simulink model "EcoSIM3_P2_C2_WIP"  (R2014b)
settings: Solver=ode1  SolverMode=SingleTasking  StartTime=0.0  StopTime=inf  FixedStep=0.01  RelTol=1e-3
PostLoadFcn:
  | %, if any(exist('dsrtsu_mdlpostloadfcn', 'file') == [2, 3, 6]), try dsrtsu_mdlpostloadfcn('Execute', bdroot); catch fprintf('Error in PostLoadFcn (dsrtsu_mdlpostloadfcn) for model "%s":\n %s\n', bdroot, lasterr); end, end,
InitFcn:
  | tic
  | %Startup_EcoSIM
values from neighbouring files (symbols this model uses):
  EngPwr = [0 5	10	15	20	25	30	35	40	45	50	55	60	65	70	75	80	85	90	95	100	105	110	115]    [Series_Maps.m]
  EngSpd = [0 477.4645 954.929 1909.858 2864.787 3819.716 4774.645 5729.574 6684.503]    [Series_Maps.m]
  EngTrq = [0	0	0	0	0	0	0	0	0	0	0	0	0	0	0	0	0	0	0	0	0	0	0	0 ... (first row only)    [Series_Maps.m]
  Power = [0 5 10 15 20 25 30]    [Series_Maps.m]
  Torque = [-50,-40,-30,-25,-20,-15,-10,-8,-6,-4,-2,0]    [Series_Maps.m]
undefined symbols (not defined in the file or in its folder): canChannel, Controls, DriveCycles, Driver, EM_EFF_MAP, EM_PwrLoss_MAP, Glbl, Overwritten_Mode, Plants, sigbuilder_block, Trialmap, Veh_Dynamics
libraries: simulink x141, canmsglib x113, fl_lib x104, canlib x89, nesl_utility x56, sdl_lib x29, dspsigops x6, dspswit3 x5, dspstat3 x2, commnoisgen2 x1, dspfdesign x1
(part 3 of 21)

== system EcoSIM3_P2_C2_WIP/Powertrain/Accessories Power Module/Plant ==
  Actuator_Cmds : Inport
  Bus Creator1 : BusCreator  Inputs=2
  Bus Creator2 : BusCreator  Inputs=2
  Bus Creator3 : BusCreator  Inputs=3
  Bus Selector : BusSelector  OutputSignals=Accessories_Power_In_W,AccPwrMdlLowVlt,Accessories_Power_In_W,bcm_vbat
  Chart : Stateflow chart  Commented=on  TreatAsAtomicUnit=on
  Constant : Constant  Value=0
  Constant1 : Constant  Value=0
  Constant2 : Constant  Value=25
  Constant3 : Constant  Value=25
  Constant4 : Constant  Value=0
  DCDC_Eff : Gain  Gain=1/Plants.DCDC.Eff
  Data Type Conversion2 : DataTypeConversion  OutDataTypeStr=boolean
  Divide : Product  Inputs=*/
  Divide1 : Product  Inputs=*/
  Saturation1 : Saturate  UpperLimit=255  LowerLimit=0
  Switch : Switch  Criteria=u2 > Threshold
  Switch1 : Switch  Criteria=u2 > Threshold
  Sensor_Out : Outport
  tag scope: DCDC_HV_Crnt=global
  wires:
  Constant4/1 -> Data Type Conversion2/1
  Data Type Conversion2/1 -> Bus Creator3/3  "Fault"
  Constant3/1 -> Bus Creator3/2  "AccPwrModTmp2"
  Constant2/1 -> Bus Creator3/1  "AccPwrModTmp1"
  Bus Creator3/1 -> Bus Creator2/1  "Temperature_Sensors"
  Bus Creator1/1 -> Bus Creator2/2  "Electrical_Sensors"
  Bus Creator2/1 -> Sensor_Out/1  "APM_Sensor_Out"
  Actuator_Cmds/1 -> Bus Selector/1
  Bus Selector/2 -> Divide/2, Switch/2  "<AccPwrMdlLowVlt>"
  Switch/1 -> Bus Creator1/1  "APMLwVltOtptCrntUns"
  Bus Selector/1 -> Divide/1  "<Accessories_Power_In_W>"
  Bus Selector/4 -> Divide1/2, Switch1/2  "<bcm_vbat>"
  Switch1/1 -> [DCDC_HV_Crnt], Bus Creator1/2  "AccPwrMdlHiVltInpCrnt"
  Divide/1 -> Saturation1/1
  Saturation1/1 -> Switch/1
  Constant/1 -> Switch/3
  Divide1/1 -> DCDC_Eff/1
  DCDC_Eff/1 -> Switch1/1
  Constant1/1 -> Switch1/3
  Bus Selector/3 -> Divide1/1  "<Accessories_Power_In_W>"

== system EcoSIM3_P2_C2_WIP/Powertrain/Accessories Power Module/Subsystem ==
  CAN_In : Inport
  Sensor_In : Inport  Port=2
  Algorithm : Subsystem
  Inputs : Subsystem
  Outputs : Subsystem
  To ECU : Outport
  Actuator_Cmds : Outport  Port=2
  wires:
  CAN_In/1 -> Inputs/1(CAN_In)  "APM_CAN_In"
  Algorithm/1(Outputs) -> Outputs/1(From Algorithm)
  Sensor_In/1 -> Inputs/2(Sensors)
  Inputs/1(To_Algorithm) -> Algorithm/1(Inputs)
  Outputs/1(To ECU) -> To ECU/1
  Outputs/2(Actuator_Cmds) -> Actuator_Cmds/1

== system EcoSIM3_P2_C2_WIP/Powertrain/BAS Motor/ Compnent Model ==
  Actuator_Cmds : Inport
  Actuators : Subsystem
  Plant : Subsystem
  Sensors : Subsystem
  To_Plants : PMIOPort  Port=1  Side=Right
  Sensor_Out : Outport
  To_Battery : Outport  Port=2
  wires:
  Actuator_Cmds/1 -> Actuators/1(ActuatorInputs)
  Actuators/1(Actuator Outputs) -> Plant/1(From_Actuators)
  Sensors/1(Sensor Out) -> Sensor_Out/1, Plant/2(Sensor_Feedback)  "BAS_Sensor_Out"
  Sensors/2(Battery) -> To_Battery/1
  connections:
  To_Plants/RConn1 -- Sensors/RConn1
  Plant/RConn1 -- Sensors/LConn1

== system EcoSIM3_P2_C2_WIP/Powertrain/BAS Motor/BAS_Receive ==
  note: Put the CAN Recieve Block placed in the
      | Vehicle Network ToolBox and define the
      | Messages required
  From_ECUs : Outport
  wires:
  [BAS_SoftECU_Receive] -> From_ECUs/1  "BAS_SoftECU_Receive"

== system EcoSIM3_P2_C2_WIP/Powertrain/BAS Motor/BAS_Transmit ==
  note: Put the CAN Transmit Block placed in the
      | Vehicle Network ToolBox and define the
      | Messages required
  To_ECUs : Inport
  Bus Creator{,1,3..4} (4 alike) : BusCreator  Inputs=2
  Bus Creator2 : BusCreator  Inputs=3
  Bus Selector : BusSelector  OutputSignals=BAS_Speed_rad_per_s,BAS_Torque_Out_Nm,BAS_Torque_Command_Nm,BAS_Status_Mode,BAS_Fault_Status,Fault_U,Fault_V,Fault_W
  Ground : Ground
  Ground1 : Ground
  Terminator : Terminator
  Terminator1 : Terminator
  Terminator2 : Terminator
  tag scope: BAS_SoftECU_Transmit=global
  wires:
  Bus Creator4/1 -> [BAS_SoftECU_Transmit]  "BAS_Transmit"
  To_ECUs/1 -> Bus Selector/1
  Bus Selector/6 -> Bus Creator2/1  "<Fault_U>"
  Bus Selector/3 -> Terminator/1  "<BAS_Torque_Command_Nm>"
  Bus Selector/8 -> Bus Creator2/3  "<Fault_W>"
  Bus Selector/1 -> Bus Creator1/1  "<BAS_Speed_rad_per_s>"
  Bus Selector/4 -> Terminator1/1  "<BAS_Status_Mode>"
  Bus Selector/7 -> Bus Creator2/2  "<Fault_V>"
  Bus Selector/5 -> Terminator2/1  "<BAS_Fault_Status>"
  Bus Creator1/1 -> Bus Creator/1  "Status_1"
  Bus Selector/2 -> Bus Creator1/2  "<BAS_Torque_Out_Nm>"
  Bus Creator2/1 -> Bus Creator/2  "Status_2"
  Bus Creator/1 -> Bus Creator4/1  "BAS_CAN_Out"
  Bus Creator3/1 -> Bus Creator4/2  "BAS_Electrical_Out"
  Ground1/1 -> Bus Creator3/2  "Dummy2"
  Ground/1 -> Bus Creator3/1  "Dummy1"

== system EcoSIM3_P2_C2_WIP/Powertrain/BAS Motor/Soft ECU ==
  CAN_In : Inport
  Sensor_In : Inport  Port=2
  Algorithm : Subsystem
  Inputs : Subsystem
  Inputs1 : Subsystem
  CAN_Out : Outport
  Actuator_Cmds : Outport  Port=2
  wires:
  Sensor_In/1 -> Inputs/2(Sensors)
  CAN_In/1 -> Inputs/1(CAN_In)
  Inputs/1(To_Algorithm) -> Algorithm/1(Inputs)
  Algorithm/1(Outputs) -> Inputs1/1(From Algorithm)
  Inputs1/1(CAN Out) -> CAN_Out/1
  Inputs1/2(Actuator Cmds) -> Actuator_Cmds/1

== system EcoSIM3_P2_C2_WIP/Powertrain/Belt Coupler/Sensors ==
  note: Sensor Model: Place where we add Corrupter
  Ideal Rotational Motion Sensor : fl_lib/Mechanical/Mechanical Sensors/Ideal Rotational Motion Sensor  offset=0 rad
  Ideal Torque Sensor : fl_lib/Mechanical/Mechanical Sensors/Ideal Torque Sensor
  Mechanical Rotational Reference1 : fl_lib/Mechanical/Rotational Elements/Mechanical Rotational Reference
  PS-Simulink Converter : nesl_utility/PS-Simulink Converter  PhysicalDomain=network_engine_domain  SubClassName=ps_output  LeftPortType=input  RightPortType=output  PseudoPeriodic=off  Frequencies=[]  Unit=rad/s  AffineConversion=off
  PS-Simulink Converter1 : nesl_utility/PS-Simulink Converter  PhysicalDomain=network_engine_domain  SubClassName=ps_output  LeftPortType=input  RightPortType=output  PseudoPeriodic=off  Frequencies=[]  Unit=N*m  AffineConversion=off
  Terminator : Terminator
  Terminator1 : Terminator
  Shaft : PMIOPort  Port=1  Side=Left
  To_Clutch : PMIOPort  Tag=PMCPort  Port=2  Side=Right
  wires:
  PS-Simulink Converter/1 -> Terminator/1  "Belt_Speed_rad_per_s"
  PS-Simulink Converter1/1 -> Terminator1/1  "Belt_Torque_Out_Nm"
  connections:
  Ideal Torque Sensor/LConn1 -- Shaft/RConn1 -- Ideal Rotational Motion Sensor/LConn1
  Ideal Rotational Motion Sensor/RConn1 -- Mechanical Rotational Reference1/LConn1
  PS-Simulink Converter/LConn1 -- Ideal Rotational Motion Sensor/RConn2
  PS-Simulink Converter1/LConn1 -- Ideal Torque Sensor/RConn2
  To_Clutch/RConn1 -- Ideal Torque Sensor/RConn1

== system EcoSIM3_P2_C2_WIP/Powertrain/Charger/CAN_Revieve ==
  note: Put the CAN Recieve Block placed in the
      | Vehicle Network ToolBox and define the
      | Messages required
  Bus Selector : BusSelector  OutputSignals=Brusa_Electrical.PON
  From_ECUs : Outport
  wires:
  [Brusa_SoftECU_Receive] -> Bus Selector/1
  Bus Selector/1 -> From_ECUs/1  "<PON>"

== system EcoSIM3_P2_C2_WIP/Powertrain/Charger/CAN_Transmit ==
  note: Put the CAN Transmit Block placed in the
      | Vehicle Network ToolBox and define the
      | Messages required
  To_CAN : Inport
  Bus Creator : BusCreator  Inputs=1
  Bus Creator1 : BusCreator  Inputs=2
  Bus Creator3 : BusCreator  Inputs=1
  Bus Creator4 : BusCreator  Inputs=2
  Bus Selector : BusSelector  OutputSignals=chga_wake,GCM_Wakeup_charge
  Ground : Ground
  Ground1 : Ground
  Terminator : Terminator
  tag scope: Brusa_SoftECU_Transmit=global
  wires:
  To_CAN/1 -> Bus Selector/1
  Bus Creator/1 -> Bus Creator4/1  "Brusa_CAN_Out"
  Bus Creator1/1 -> Bus Creator/1  "Brusa_Dummy_msg"
  Bus Creator3/1 -> Bus Creator4/2  "Brusa_Electrical_Out"
  Bus Creator4/1 -> [Brusa_SoftECU_Transmit]  "Brusa_Transmit"
  Ground1/1 -> Bus Creator1/1  "Dummy1"
  Ground/1 -> Bus Creator1/2  "Dummy2"
  Bus Selector/1 -> Terminator/1  "<chga_wake>"
  Bus Selector/2 -> Bus Creator3/1  "<GCM_Wakeup_charge>"

== system EcoSIM3_P2_C2_WIP/Powertrain/Charger/Plant ==
  FromSoftECU : Inport
  Gain : Gain  Gain=-3300
  To Plant : Outport
  wires:
  FromSoftECU/1 -> Gain/1
  Gain/1 -> To Plant/1

== system EcoSIM3_P2_C2_WIP/Powertrain/Charger/Soft ECU ==
  FromESS : Inport
  AC : Inport  Port=2
  Algorithm : Subsystem
  Inputs : Subsystem
  Outputs : Subsystem
  ToECUs : Outport
  Actuator_Cmds : Outport  Port=2
  wires:
  Algorithm/1(Outputs) -> Outputs/1(From Algorithm)
  Inputs/1(To_Algorithm) -> Algorithm/1(Inputs)
  Outputs/1(ToECUs) -> ToECUs/1
  AC/1 -> Inputs/2(Supply)
  FromESS/1 -> Inputs/1(FromESS1)
  Outputs/2(Actuator_Cmds) -> Actuator_Cmds/1

== system EcoSIM3_P2_C2_WIP/Powertrain/Clutch_Transmission1/CAN_Recieve ==
  note: Put the CAN Recieve Block placed in the
      | Vehicle Network ToolBox and define the
      | Messages required
  Bus Creator : BusCreator  Inputs=1
  From_CAN : Outport
  wires:
  Bus Creator/1 -> From_CAN/1
  [Clutch_Trans_SoftECU_Receive] -> Bus Creator/1  "Clutch_Trans_SoftECU_Receive"

== system EcoSIM3_P2_C2_WIP/Powertrain/Clutch_Transmission1/CAN_Transmit ==
  note: Put the CAN Transmit Block placed in the
      | Vehicle Network ToolBox and define the
      | Messages required
  To_CAN : Inport
  Bus Creator : BusCreator  Inputs=1
  Bus Creator1 : BusCreator  Inputs=2
  Bus Creator2 : BusCreator  Inputs=2
  Ground : Ground
  Ground1 : Ground
  tag scope: Clutch_Trans_SoftECU_Transmit=global
  wires:
  Bus Creator1/1 -> [Clutch_Trans_SoftECU_Transmit]  "Clutch_Transmission_SoftECU_Transmit"
  Ground1/1 -> Bus Creator2/2  "Dummy2"
  Ground/1 -> Bus Creator2/1  "Dummy1"
  Bus Creator2/1 -> Bus Creator1/2  "Clutch_Transmission_Electrical_Out"
  Bus Creator/1 -> Bus Creator1/1  "Clutch_Transmission_CAN_Out"
  To_CAN/1 -> Bus Creator/1

== system EcoSIM3_P2_C2_WIP/Powertrain/Clutch_Transmission1/CP1 SoftEcu ==
  From GCM : Inport
  Sensor_In : Inport  Port=2
  Algorithm : Subsystem
  Inputs : Subsystem
  Inputs1 : Subsystem
  To_GCM : Outport
  Actuator_Cmds : Outport  Port=2
  wires:
  Inputs1/2(To GCM) -> To_GCM/1
  Inputs1/1(Actuator Cmd) -> Actuator_Cmds/1
  Algorithm/1(Outputs) -> Inputs1/1(From Algorithm)
  Sensor_In/1 -> Inputs/1(Sensors)  "Component_Sensor_Out"
  From GCM/1 -> Inputs/2(From GCM)  "Component_CAN_In"
  Inputs/1(To_Algorithm) -> Algorithm/1(Inputs)

== system EcoSIM3_P2_C2_WIP/Powertrain/Clutch_Transmission1/Clutch_Plant ==
  note: The physical signal output M corresponds to the clutch mode, and
      | equals -1 for negative slip, 0 if locked, and +1 for positive slip.
  Clutch_Engage : Inport
  Bus Selector : BusSelector  OutputSignals=Clutch_Trans_SoftECU_Receive.Clutch_Trans_CAN.Trans_Receive.Shift_Request
  Constant1 : Constant  Value=4400000
  Custom Clutch : Subsystem  Commented=on  DialogController=PMDialogs.PMDefaultMaskDlg
  Disk Friction Clutch : sdl_lib/Clutches/Disk Friction Clutch  geometry_model=1  r_eff=130 mm  d_o=150 mm  d_i=100 mm  nS=4  piston_area=0.001 m^2  unidirectional=0  friction_model=1  mu_coulomb=0.3  mu_w_vector=[ 0 0.1 0.2 0.3 0.4 0.5 1 2 5 10 100 1000 ] rad/s  mu_coulomb_vector=[ 0.29 0.28 0.26 0.22 0.21 0.2 0.2 0.19 0.19 0.19 0.19 0.19 ]  mu_interp_method=1  mu_extrap_method=1  mu_static=0.35  d_f=1  w_tol=0.001 rad/s  pressure_min=100 Pa  mu_visc=0 N*m/(rad/s)  initial_state_locked=0
      settings: LogSimulationData=on
  Gain : Gain  Gain=0.4
  IC : InitialCondition  Value=0
  Inertia1 : fl_lib/Mechanical/Rotational Elements/Inertia  inertia=0.01 kg*m^2  w_specify=off  w_priority=High  w=0 rad/s  t_specify=off  t_priority=High  t=0 N*m
  Product : Product
  Rate Limiter : RateLimiter  SampleTimeMode=inherited
  Scope : Scope
      settings: SaveName=ScopeData33
  Sensors : Subsystem
  Simulink-PS Converter1 : nesl_utility/Simulink-PS Converter  PhysicalDomain=network_engine_domain  SubClassName=ps_input  LeftPortType=input  RightPortType=output  PseudoPeriodic=off  Frequencies=[]  NoiseDistribution=none  NoiseParameters=[]  Unit=Pa  AffineConversion=off  InputFiltering=off  SimscapeFilterOrder=1  InputFilterTimeConstant=.001  UdotUserProvided=1
  Terminator : Terminator
  Terminator1 : Terminator
  ToTrans : PMIOPort  Port=1  Side=Right
  ICE Output Shaft : PMIOPort  Tag=PMCPort  Port=2  Side=Left
  Clutch_Status : Outport
  wires:
  IC/1 -> Terminator1/1  "Shift_Request_Clutch"
  Gain/1 -> Product/1
  Rate Limiter/1 -> Product/2, Scope/1
  Constant1/1 -> Gain/1
  Product/1 -> Simulink-PS Converter1/1, Sensors/1(Clutch_Pressure)  "Clutch_Pressure_Pa"
  Clutch_Engage/1 -> Terminator/1, Bus Selector/1
  Bus Selector/1 -> IC/1, Rate Limiter/1  "<Shift_Request>"
  Sensors/1(Clutch_Status) -> Clutch_Status/1
  connections:
  Disk Friction Clutch/LConn1 -- Simulink-PS Converter1/RConn1
  Disk Friction Clutch/RConn1 -- Inertia1/LConn1 -- Sensors/LConn1
  ToTrans/RConn1 -- Sensors/RConn1
  ICE Output Shaft/RConn1 -- Disk Friction Clutch/LConn2

== system EcoSIM3_P2_C2_WIP/Powertrain/Clutch_Transmission1/GCM ==
  CAN_In : Inport
  From CP1 : Inport  Port=2
  GCM Soft ECU : Subsystem
  Inputs : Subsystem
  Outputs : Subsystem
  CAN Out : Outport
  To SoftECU : Outport  Port=2
  wires:
  GCM Soft ECU/1(Outputs) -> Outputs/1(From Algorithm)
  Outputs/2(To_SoftECU) -> To SoftECU/1
  Outputs/1(CAN_Out) -> CAN Out/1
  Inputs/1(To_Algorithm) -> GCM Soft ECU/1(Inputs)
  CAN_In/1 -> Inputs/2(CAN_In)
  From CP1/1 -> Inputs/1(From SoftECU)

== system EcoSIM3_P2_C2_WIP/Powertrain/Clutch_Transmission1/Mastershift Softecu ==
  From GCM : Inport
  Clutch_CAN_Out : Inport  Port=2
  Sensor_In : Inport  Port=3
  Algorithm : Subsystem
  Inputs : Subsystem
  Outputs : Subsystem
  To_GCM : Outport
  Actuator_Cmds : Outport  Port=2
  wires:
  Outputs/2(To GCM) -> To_GCM/1
  Outputs/1(Actuator Commands) -> Actuator_Cmds/1
  Algorithm/1(Outputs) -> Outputs/1(From Algorithm)
  Clutch_CAN_Out/1 -> Inputs/3(Clutch_CAN_Out)
  Inputs/1(To_Algorithm) -> Algorithm/1(Inputs)
  From GCM/1 -> Inputs/2(From GCM)
  Sensor_In/1 -> Inputs/1(Sensors)

== system EcoSIM3_P2_C2_WIP/Powertrain/Clutch_Transmission1/Trans_Plant ==
  Gear_Cmd : Inport
  Actuators : Subsystem
  Plant : Subsystem
  Sensors : Subsystem
  Trans Input Shaft : PMIOPort  Port=1  Side=Left
  Trans Output Shaft : PMIOPort  Port=2  Side=Right
  Sensor_Out : Outport
  ActGear : Outport  Port=2
  wires:
  Sensors/2(ActGear) -> ActGear/1
  Plant/1(Actual_Gear) -> Sensors/1(Actual_Gear)
  Gear_Cmd/1 -> Actuators/1(ActuatorInputs)
  Actuators/1(Actuator Outputs) -> Plant/1(From_Actuators)
  Sensors/1(Sensor Out) -> Sensor_Out/1  "Trans_Sensor_Out"
  connections:
  Trans Input Shaft/RConn1 -- Plant/LConn1
  Trans Output Shaft/RConn1 -- Sensors/RConn1
  Plant/RConn1 -- Sensors/LConn1

== system EcoSIM3_P2_C2_WIP/Powertrain/Clutch_Transmission2/CAN_Recieve ==
  note: Put the CAN Recieve Block placed in the
      | Vehicle Network ToolBox and define the
      | Messages required
  Bus Creator : BusCreator  Inputs=2
  From_CAN : Outport
  wires:
  Bus Creator/1 -> From_CAN/1
  [CP1_SoftECU_Receive] -> Bus Creator/1  "CP1_SoftECU_Receive"
  [Mastershift_SoftECU_Receive] -> Bus Creator/2  "Mastershift_SoftECU_Receive"

== system EcoSIM3_P2_C2_WIP/Powertrain/Clutch_Transmission2/CAN_Transmit ==
  CP1 : Inport
  MShift : Inport  Port=2
  Bus Creator{4,6..8,10} (5 alike) : BusCreator  Inputs=1
  Bus Creator3 : BusCreator  Inputs=2
  Bus Creator5 : BusCreator  Inputs=2
  Bus Creator9 : BusCreator  Inputs=2
  Bus Selector : BusSelector  OutputSignals=CY01_stMode,CY01_posCurr,Dummy_Electrical1
  Bus Selector1 : BusSelector  OutputSignals=Dummy_Electrical1,Mastershift_Gear
  tag scope: CP1_SoftECU_Transmit=global, Mastershift_SoftECU_Transmit=global
  wires:
  CP1/1 -> Bus Selector/1
  Bus Selector/2 -> Bus Creator3/2  "<CY01_posCurr>"
  Bus Selector/1 -> Bus Creator3/1  "<CY01_stMode>"
  Bus Creator3/1 -> Bus Creator4/1  "CCU_HYB_01"
  Bus Creator4/1 -> Bus Creator5/1  "CP1_CAN_Out"
  Bus Selector/3 -> Bus Creator6/1  "<Dummy_Electrical1>"
  Bus Creator6/1 -> Bus Creator5/2  "CP1_Electrical_Out"
  Bus Creator5/1 -> [CP1_SoftECU_Transmit]  "CP1_Transmit"
  MShift/1 -> Bus Selector1/1
  Bus Selector1/2 -> Bus Creator10/1  "<Mastershift_Gear>"
  Bus Creator7/1 -> Bus Creator8/1  "Message_01"
  Bus Creator8/1 -> Bus Creator9/1  "Mastershift_CAN_Out"
  Bus Creator10/1 -> Bus Creator9/2  "Mastershift_Electrical_Out"
  Bus Creator9/1 -> [Mastershift_SoftECU_Transmit]  "Mastershift_Transmit"
  Bus Selector1/1 -> Bus Creator7/1  "<Dummy_Electrical1>"

== system EcoSIM3_P2_C2_WIP/Powertrain/Clutch_Transmission2/CP1 SoftEcu ==
  CANRx : Inport
  Sensor_In : Inport  Port=2
  Algorithm : Subsystem
  Inputs : Subsystem
  Outputs : Subsystem
  CANTx : Outport
  Actuator_Cmds : Outport  Port=2
  wires:
  Inputs/1(To_Algorithm) -> Algorithm/1(Inputs)
  CANRx/1 -> Inputs/2(CAN)  "Component_CAN_In"
  Sensor_In/1 -> Inputs/1(Sensors)  "Component_Sensor_Out"
  Algorithm/1(Outputs) -> Outputs/1(From Algorithm)
  Outputs/1(Actuator Cmd) -> Actuator_Cmds/1
  Outputs/2(CAN) -> CANTx/1

== system EcoSIM3_P2_C2_WIP/Powertrain/Clutch_Transmission2/Clutch_Plant ==
  note: Engagement piston area changed from
      | 0.001 to 0.01 sq.m
  note: The physical signal output M corresponds to the clutch mode, and
      | equals -1 for negative slip, 0 if locked, and +1 for positive slip.
  Clutch_Engage : Inport
  Add : Sum  Inputs=-+
  Bus Selector : BusSelector  OutputSignals=SpA_Position_Command
  Constant : Constant
  Constant1 : Constant  Value=4400000
  Custom Clutch : Subsystem  Commented=on  DialogController=PMDialogs.PMDefaultMaskDlg
  Disk Friction Clutch : sdl_lib/Clutches/Disk Friction Clutch  geometry_model=1  r_eff=130 mm  d_o=150 mm  d_i=100 mm  nS=4  piston_area=0.001 m^2  unidirectional=0  friction_model=1  mu_coulomb=0.3  mu_w_vector=[ 0 0.1 0.2 0.3 0.4 0.5 1 2 5 10 100 1000 ] rad/s  mu_coulomb_vector=[ 0.29 0.28 0.26 0.22 0.21 0.2 0.2 0.19 0.19 0.19 0.19 0.19 ]  mu_interp_method=1  mu_extrap_method=1  mu_static=0.35  d_f=1  w_tol=0.001 rad/s  pressure_min=100 Pa  mu_visc=0 N*m/(rad/s)  initial_state_locked=0
      settings: LogSimulationData=on
  Gain : Gain  Gain=0.4
  Inertia1 : fl_lib/Mechanical/Rotational Elements/Inertia  inertia=0.01 kg*m^2  w_specify=off  w_priority=High  w=0 rad/s  t_specify=off  t_priority=High  t=0 N*m
  Product : Product
  Rate Limiter : RateLimiter  RisingSlewLimit=20  FallingSlewLimit=-8  SampleTimeMode=inherited
  Scope : Scope
      settings: SaveName=ScopeData33
  Scope1 : Scope
      settings: SaveName=ScopeData42
  Sensors : Subsystem
  Simulink-PS Converter1 : nesl_utility/Simulink-PS Converter  PhysicalDomain=network_engine_domain  SubClassName=ps_input  LeftPortType=input  RightPortType=output  PseudoPeriodic=off  Frequencies=[]  NoiseDistribution=none  NoiseParameters=[]  Unit=Pa  AffineConversion=off  InputFiltering=off  SimscapeFilterOrder=1  InputFilterTimeConstant=.001  UdotUserProvided=1
  Terminator : Terminator
  ToTrans : PMIOPort  Port=1  Side=Right
  ICE Output Shaft : PMIOPort  Tag=PMCPort  Port=2  Side=Left
  Clutch_Status : Outport
  wires:
  Sensors/1(Clutch_Status) -> Clutch_Status/1
  Bus Selector/1 -> Scope1/1, Add/1  "<SpA_Position_Command>"
  Clutch_Engage/1 -> Bus Selector/1, Terminator/1
  Product/1 -> Sensors/1(Clutch_Pressure), Simulink-PS Converter1/1  "Clutch_Pressure_Pa"
  Constant1/1 -> Gain/1
  Gain/1 -> Product/1
  Constant/1 -> Add/2
  Add/1 -> Rate Limiter/1
  Rate Limiter/1 -> Product/2, Scope/1
  connections:
  ICE Output Shaft/RConn1 -- Disk Friction Clutch/LConn2
  ToTrans/RConn1 -- Sensors/RConn1
  Sensors/LConn1 -- Inertia1/LConn1 -- Disk Friction Clutch/RConn1
  Disk Friction Clutch/LConn1 -- Simulink-PS Converter1/RConn1

== system EcoSIM3_P2_C2_WIP/Powertrain/Clutch_Transmission2/Mastershift Softecu ==
  CANRx : Inport
  Sensor_In : Inport  Port=2
  Algorithm : Subsystem
  Inputs : Subsystem
  Outputs : Subsystem
  CANTx : Outport
  Actuator_Cmds : Outport  Port=2
  wires:
  Sensor_In/1 -> Inputs/1(Sensors)
  CANRx/1 -> Inputs/2(CAN)
  Inputs/1(To_Algorithm) -> Algorithm/1(Inputs)
  Algorithm/1(Outputs) -> Outputs/1(From Algorithm)
  Outputs/1(Actuator Commands) -> Actuator_Cmds/1
  Outputs/2(CANTx) -> CANTx/1

== system EcoSIM3_P2_C2_WIP/Powertrain/Clutch_Transmission2/Trans_Plant ==
  Gear_Cmd : Inport
  Actuators : Subsystem
  Plant : Subsystem
  Sensors : Subsystem
  Trans Input Shaft : PMIOPort  Port=1  Side=Left
  Trans Output Shaft : PMIOPort  Port=2  Side=Right
  Sensor_Out : Outport
  wires:
  Sensors/1(Sensor Out) -> Sensor_Out/1  "Trans_Sensor_Out"
  Actuators/1(Actuator Outputs) -> Plant/1(From_Actuators)
  Gear_Cmd/1 -> Actuators/1(ActuatorInputs)
  Plant/1(Actual_Gear) -> Sensors/1(Actual_Gear)
  connections:
  Plant/RConn1 -- Sensors/LConn1
  Trans Output Shaft/RConn1 -- Sensors/RConn1
  Trans Input Shaft/RConn1 -- Plant/LConn1

== system EcoSIM3_P2_C2_WIP/Powertrain/Electric Motor / Component Model ==
  Actuator_Cmds : Inport
  Actuators : Subsystem
  Plant : Subsystem
  Sensors : Subsystem
  To_Plants : PMIOPort  Port=1  Side=Right
  Sensor_Out : Outport
  To_Battery : Outport  Port=2
  wires:
  Actuator_Cmds/1 -> Actuators/1(ActuatorInputs)
  Actuators/1(Actuator Outputs) -> Plant/1(From_Actuators)
  Plant/1(To_Sensors) -> Sensors/1(Sensor In)
  Sensors/1(Sensor Out) -> Sensor_Out/1, Plant/2(Sensor_Feedback)  "EM_Sensor_Out"
  Sensors/2(To_Battery) -> To_Battery/1
  connections:
  Sensors/LConn1 -- Plant/RConn1
  Sensors/RConn1 -- To_Plants/RConn1

== system EcoSIM3_P2_C2_WIP/Powertrain/Electric Motor /EM_Receive ==
  note: Put the CAN Recieve Block placed in the
      | Vehicle Network ToolBox and define the
      | Messages required
  Bus Creator : BusCreator  Inputs=2
  From_ECUs : Outport
  wires:
  Bus Creator/1 -> From_ECUs/1
  [EM_SoftECU_Receive] -> Bus Creator/1  "EM_CAN_Messages"
  [ESS_SoftECU_Transmit] -> Bus Creator/2

== system EcoSIM3_P2_C2_WIP/Powertrain/Electric Motor /EM_Transmit ==
  note: Put the CAN Transmit Block placed in the
      | Vehicle Network ToolBox and define the
      | Messages required
  To_ECUs : Inport
  Bus Creator : BusCreator  Inputs=7
  Bus Creator{1..2,8..9} (4 alike) : BusCreator  Inputs=1
  Bus Creator3 : BusCreator  Inputs=3
  Bus Creator4 : BusCreator  Inputs=2
  Bus Creator5 : BusCreator  Inputs=2
  Bus Creator6 : BusCreator  Inputs=2
  Bus Creator7 : BusCreator
  Bus Selector : BusSelector  OutputSignals=Status.Motor_Speed,Status.EM_Torque_Out_Nm,Status.Inverter_Enable_Lockout,Status.VSM_State,Status.Direction_Command_Feedback,RunningStatus.RUN_Fault,Status.POST_Fault,Status.Temperatures.Module_A,Status.Temperatures.Module_B,Status.Temperatures.Module_C,Status.Temperatures.Gate_Driver_Board,Status.Temperatures.Control_Board_Temperature,Status.Temperatures.Motor_Temperature
  Ground : Ground
  Ground1 : Ground
  tag scope: EM_SoftECU_Transmit=global
  wires:
  To_ECUs/1 -> Bus Selector/1
  Bus Creator4/1 -> [EM_SoftECU_Transmit]  "EM_Transmit"
  Bus Selector/1 -> Bus Creator1/1  "<Motor_Speed>"
  Bus Selector/6 -> Bus Creator6/1  "<RUN_Fault>"
  Bus Selector/3 -> Bus Creator3/1  "<Inverter_Enable_Lockout>"
  Bus Selector/2 -> Bus Creator2/1  "<EM_Torque_Out_Nm>"
  Bus Creator1/1 -> Bus Creator/1  "M165_Motor_Position_Info"
  Bus Creator2/1 -> Bus Creator/2  "M172_Torque_And_Timer_Info"
  Bus Creator3/1 -> Bus Creator/3  "M170_Internal_States"
  Bus Creator/1 -> Bus Creator4/1  "EM_CAN_Out"
  Bus Creator5/1 -> Bus Creator4/2  "EM_Electrical_Out"
  Ground/1 -> Bus Creator5/1  "Dummy1"
  Ground1/1 -> Bus Creator5/2  "Dummy2"
  Bus Selector/7 -> Bus Creator6/2  "<POST_Fault>"
  Bus Creator6/1 -> Bus Creator/4  "M171_Fault_Codes"
  Bus Selector/4 -> Bus Creator3/2  "<VSM_State>"
  Bus Selector/8 -> Bus Creator7/1  "<Module_A>"
  Bus Selector/9 -> Bus Creator7/2  "<Module_B>"
  Bus Selector/10 -> Bus Creator7/3  "<Module_C>"
  Bus Selector/11 -> Bus Creator7/4  "<Gate_Driver_Board>"
  Bus Selector/12 -> Bus Creator8/1  "<Control_Board_Temperature>"
  Bus Selector/13 -> Bus Creator9/1  "<Motor_Temperature>"
  Bus Creator7/1 -> Bus Creator/5  "M160_Temperature_Set_1"
  Bus Creator8/1 -> Bus Creator/6  "M161_Temperature_Set_2"
  Bus Creator9/1 -> Bus Creator/7  "M162_Temperature_Set_3"
  Bus Selector/5 -> Bus Creator3/3  "<Direction_Command_Feedback>"

== system EcoSIM3_P2_C2_WIP/Powertrain/Electric Motor /Soft ECU ==
  From_ECUs : Inport
  Sensor_In : Inport  Port=2
  Algorithm : Subsystem
  Inputs : Subsystem
  Outputs : Subsystem
  To_ECUs : Outport
  Actuator_Cmds : Outport  Port=2
  wires:
  Sensor_In/1 -> Inputs/2(Sensors)
  From_ECUs/1 -> Inputs/1(From_ECUs)
  Inputs/1(To_Algorithm) -> Algorithm/1(Inputs)
  Algorithm/1(Outputs) -> Outputs/1(From Algorithm)
  Outputs/1(To_ECUs) -> To_ECUs/1
  Outputs/2(Actuator Commands) -> Actuator_Cmds/1

== system EcoSIM3_P2_C2_WIP/Powertrain/Electrical Storage System/ ESS Model ==
  Actuator_Cmds : Inport
  Charger_Power_In [W] : Inport  Port=2
  EM_Power_In [W] : Inport  Port=3
  Accessories_Power_In [W] : Inport  Port=4
  BAS_Power_In [W] : Inport  Port=5
  Actuators : Subsystem
  Plant : Subsystem
  Sensors : Subsystem
  Sensor_Out : Outport
  wires:
  Actuator_Cmds/1 -> Actuators/1(ActuatorInputs)
  Actuators/1(Actuator Outputs) -> Plant/1(From_Actuators)
  Plant/1(To_Sensors) -> Sensors/1(Sensor In)
  Sensors/1(Sensor Out) -> Sensor_Out/1  "Component_Sensor_Out"
  EM_Power_In [W]/1 -> Actuators/3(EM P_in [W])
  Accessories_Power_In [W]/1 -> Actuators/4(Acc P_in [W])
  BAS_Power_In [W]/1 -> Actuators/5(BAS P_in [W])
  Charger_Power_In [W]/1 -> Actuators/2(Charger_P_in [W])

== system EcoSIM3_P2_C2_WIP/Powertrain/Electrical Storage System/CAN_Revieve ==
  note: Put the CAN Recieve Block placed in the
      | Vehicle Network ToolBox and define the
      | Messages required
  Bus Creator : BusCreator  Inputs=8
  Bus Selector : BusSelector  OutputSignals=BCM_CAN.BCM_Request.hsc_bcm_enable,BCM_CAN.BCM_Request.hsc_bcm_mainc_close,BCM_CAN.BCM_Request.hsc_bcm_leakage_ena,BCM_CAN.BCM_Request.hsc_bcm_epo,BCM_Electrical.BMS_Powerup,BCM_Electrical.chga_wake,BCM_Electrical.veh_wake
  From_CAN : Outport
  wires:
  Bus Creator/1 -> From_CAN/1
  [ESS_SoftECU_Receive] -> Bus Selector/1
  Bus Selector/1 -> Bus Creator/1  "<hsc_bcm_enable>"
  Bus Selector/2 -> Bus Creator/2  "<hsc_bcm_mainc_close>"
  Bus Selector/3 -> Bus Creator/3  "<hsc_bcm_leakage_ena>"
  Bus Selector/4 -> Bus Creator/4  "<hsc_bcm_epo>"
  Bus Selector/5 -> Bus Creator/5  "<BMS_Powerup>"
  Bus Selector/6 -> Bus Creator/6  "<chga_wake>"
  Bus Selector/7 -> Bus Creator/7  "<veh_wake>"
  [DCDC_HV_Crnt] -> Bus Creator/8

== system EcoSIM3_P2_C2_WIP/Powertrain/Electrical Storage System/CAN_Transmit ==
  note: Put the CAN Transmit Block placed in the
      | Vehicle Network ToolBox and define the
      | Messages required
  To_CAN : Inport
  Bus Creator : BusCreator
  Bus Creator1 : BusCreator  Inputs=12
  Bus Creator2 : BusCreator  Inputs=3
  Bus Creator3 : BusCreator  Inputs=1
  Bus Creator4 : BusCreator  Inputs=2
  Bus Creator5 : BusCreator  Inputs=2
  Bus Creator6 : BusCreator  Inputs=1
  Bus Selector : BusSelector  OutputSignals=bcm_chg_done,Batt_SOC_percent,bcm_ready,bcm_hvil_mon,bcm_mainc_stat,bcm_chgc_stat,bcm_cpwr_cmd,bcm_cpwr_mon,bcm_epo,Batt_Voltage_V,Batt_Current_A,bcm_on_plug,bcm_veh_mon,bcm_cell_tmax,bcm_cell_tmin,bcm_dis_buf,chga_ena
  Gain : Gain
  Gain1 : Gain
  Gain2 : Gain
  Ground1 : Ground
  Ground2 : Ground
  tag scope: ESS_SoftECU_Transmit=global
  wires:
  To_CAN/1 -> Bus Selector/1
  Bus Selector/2 -> Gain2/1  "<Batt_SOC_percent>"
  Bus Creator/1 -> Bus Creator4/1  "ESS_CAN_Out"
  Bus Selector/3 -> Bus Creator1/3  "<bcm_ready>"
  Bus Selector/4 -> Bus Creator1/4  "<bcm_hvil_mon>"
  Bus Selector/5 -> Bus Creator1/5  "<bcm_mainc_stat>"
  Bus Selector/6 -> Bus Creator1/6  "<bcm_chgc_stat>"
  Bus Selector/7 -> Bus Creator1/7  "<bcm_cpwr_cmd>"
  Bus Selector/8 -> Bus Creator1/8  "<bcm_cpwr_mon>"
  Bus Selector/9 -> Bus Creator1/9  "<bcm_epo>"
  Bus Selector/13 -> Bus Creator2/1  "<bcm_veh_mon>"
  Bus Selector/10 -> Gain/1  "<Batt_Voltage_V>"
  Bus Selector/11 -> Gain1/1  "<Batt_Current_A>"
  Gain/1 -> Bus Creator1/10  "bcm_vbat"
  Gain1/1 -> Bus Creator1/11  "bcm_ibat"
  Bus Creator1/1 -> Bus Creator/1  "BCM_Status"
  Bus Creator2/1 -> Bus Creator/2  "BCM_Data1"
  Bus Selector/12 -> Bus Creator1/12  "<bcm_on_plug>"
  Bus Selector/17 -> Bus Creator3/1  "<chga_ena>"
  Bus Creator3/1 -> Bus Creator4/2  "ESS_Electrical_Out"
  Bus Creator4/1 -> [ESS_SoftECU_Transmit]  "ESS_Transmit"
  Gain2/1 -> Bus Creator1/2  "bcm_soc"
  Bus Selector/16 -> Bus Creator5/1  "<bcm_dis_buf>"
  Ground1/1 -> Bus Creator5/2  "bcm_chg_buf"
  Bus Creator5/1 -> Bus Creator/3  "BCM_Limits"
  Bus Selector/14 -> Bus Creator2/2  "<bcm_cell_tmax>"
  Bus Selector/15 -> Bus Creator2/3  "<bcm_cell_tmin>"
  Bus Selector/1 -> Bus Creator1/1  "<bcm_chg_done>"
  Bus Creator6/1 -> Bus Creator/4  "BCM_Data2"
  Ground2/1 -> Bus Creator6/1  "bcm_balancing"

== system EcoSIM3_P2_C2_WIP/Powertrain/Electrical Storage System/Soft ECU ==
  CAN_In : Inport
  Sensor_In : Inport  Port=2
  Algorithm : Subsystem
  Inputs : Subsystem
  Outputs : Subsystem
  To ECUs : Outport
  Actuator_Cmds : Outport  Port=2
  wires:
  Sensor_In/1 -> Inputs/1(Sensors)  "Component_Sensor_Out"
  CAN_In/1 -> Inputs/2(CAN_In)  "Component_CAN_In"
  Inputs/1(To_Algorithm) -> Algorithm/1(Inputs)
  Algorithm/1(Outputs) -> Outputs/1(From Algorithm)
  Outputs/1(Actuator_Cmds) -> Actuator_Cmds/1
  Outputs/2(To ECUs) -> To ECUs/1

== system EcoSIM3_P2_C2_WIP/Powertrain/Engine/ Component Model ==
  Actuator_Cmds : Inport
  Actuators : Subsystem
  Plant : Subsystem
  Sensors : Subsystem
  ICE Output Shaft : PMIOPort  Tag=PMCPort  Port=1  Side=Right
  Sensor_Out : Outport
  Fuel_Consumption : Outport  Port=2
  wires:
  Actuator_Cmds/1 -> Actuators/1(ActuatorInputs)
  Actuators/1(Actuator Outputs) -> Plant/1(From_Actuators)
  Sensors/1(Sensor Out) -> Plant/2(Sensors_Feedback), Sensor_Out/1  "ICE_Sensor_Out"
  Sensors/2(Fuel) -> Fuel_Consumption/1
  Plant/1(Fuel_Consumtion_kg_per_s) -> Sensors/1(Fuel_Consumption)
  connections:
  ICE Output Shaft/RConn1 -- Sensors/RConn1
  Plant/RConn1 -- Sensors/LConn1

== system EcoSIM3_P2_C2_WIP/Powertrain/Engine/ICE_Receive ==
  note: Put the CAN Recieve Block placed in the
      | Vehicle Network ToolBox and define the
      | Messages required
  Bus Creator : BusCreator  Inputs=1
  From_ECUs : Outport
  wires:
  Bus Creator/1 -> From_ECUs/1  "ICE_From_CAN"
  [Engine_SoftECU_Receive] -> Bus Creator/1  "ECM_SoftECU_Receive"

== system EcoSIM3_P2_C2_WIP/Powertrain/Engine/ICE_Transmit ==
  note: Put the CAN Transmit Block placed in the
      | Vehicle Network ToolBox and define the
      | Messages required
  To_ECUs : Inport
  Bus Creator : BusCreator  Inputs=1
  Bus Creator1 : BusCreator  Inputs=2
  Bus Creator2 : BusCreator  Inputs=2
  Bus Creator4 : BusCreator  Inputs=1
  Bus Selector : BusSelector  OutputSignals=ICE_Torque_Cmd_Nm
  Ground : Ground
  Ground1 : Ground
  tag scope: Engine_SoftECU_Transmit=global
  wires:
  To_ECUs/1 -> Bus Selector/1
  Bus Selector/1 -> Bus Creator/1  "<ICE_Torque_Cmd_Nm>"
  Bus Creator/1 -> Bus Creator4/1  "ICE_Torque"
  Bus Creator1/1 -> Bus Creator2/2  "ICE_Electrical_Out"
  Ground/1 -> Bus Creator1/1  "Dummy1"
  Ground1/1 -> Bus Creator1/2  "Dummy2"
  Bus Creator2/1 -> [Engine_SoftECU_Transmit]  "ICE_Transmit"
  Bus Creator4/1 -> Bus Creator2/1  "ICE_CAN_Out"

== system EcoSIM3_P2_C2_WIP/Powertrain/Engine/Soft ECU ==
  ICE_In : Inport
  Sensor_In : Inport  Port=2
  Algorithm : Subsystem
  Inputs : Subsystem
  Inputs1 : Subsystem
  ICE_Out : Outport
  Actuator_Cmds : Outport  Port=2
  wires:
  Sensor_In/1 -> Inputs/2(Sensors)
  Inputs/1(To_Algorithm) -> Algorithm/1(Inputs)
  Algorithm/1(Outputs) -> Inputs1/1(From Algorithm)
  Inputs1/1(ICE_Out) -> ICE_Out/1
  Inputs1/2(Actuator Cmds) -> Actuator_Cmds/1
  ICE_In/1 -> Inputs/1(ICE_In)

== system EcoSIM3_P2_C2_WIP/Powertrain/Mechanical Coupler/Sensors ==
  note: Sensor Model: Place where we add Corrupter
  Ideal Rotational Motion Sensor : fl_lib/Mechanical/Mechanical Sensors/Ideal Rotational Motion Sensor  offset=0 rad
  Ideal Torque Sensor : fl_lib/Mechanical/Mechanical Sensors/Ideal Torque Sensor
  Mechanical Rotational Reference1 : fl_lib/Mechanical/Rotational Elements/Mechanical Rotational Reference
  PS-Simulink Converter : nesl_utility/PS-Simulink Converter  PhysicalDomain=network_engine_domain  SubClassName=ps_output  LeftPortType=input  RightPortType=output  PseudoPeriodic=off  Frequencies=[]  Unit=rad/s  AffineConversion=off
  PS-Simulink Converter1 : nesl_utility/PS-Simulink Converter  PhysicalDomain=network_engine_domain  SubClassName=ps_output  LeftPortType=input  RightPortType=output  PseudoPeriodic=off  Frequencies=[]  Unit=N*m  AffineConversion=off
  Terminator : Terminator
  Terminator1 : Terminator
  Shaft : PMIOPort  Port=1  Side=Left
  To_Plants : PMIOPort  Port=2  Side=Right
  wires:
  PS-Simulink Converter/1 -> Terminator/1  "MC_Speed_rad_per_s"
  PS-Simulink Converter1/1 -> Terminator1/1  "MC_Torque_Out_Nm"
  connections:
  Ideal Torque Sensor/LConn1 -- Shaft/RConn1 -- Ideal Rotational Motion Sensor/LConn1
  Ideal Rotational Motion Sensor/RConn1 -- Mechanical Rotational Reference1/LConn1
  PS-Simulink Converter/LConn1 -- Ideal Rotational Motion Sensor/RConn2
  PS-Simulink Converter1/LConn1 -- Ideal Torque Sensor/RConn2
  Ideal Torque Sensor/RConn1 -- To_Plants/RConn1

== system EcoSIM3_P2_C2_WIP/Powertrain/Soft_ECUs_IO/From_Goto ==
  Bus Creator : BusCreator  Inputs=9
  Subsystem : Subsystem
  Subsystem1 : Subsystem
  Supervisory_Wakeup_Terminated : Terminator
  tag scope: BAS_SoftECU_Receive=global, Brusa_SoftECU_Receive=global, CP1_SoftECU_Receive=global, DCDC_SoftECU_Receive=global, Driver_SoftECU_Receive=global, EM_SoftECU_Receive=global, ESS_SoftECU_Receive=global, Engine_SoftECU_Receive=global, From_ECUs=global, Mastershift_SoftECU_Receive=global, Supervisory_Receive=global
  wires:
  [ESS_SoftECU_Transmit] -> Bus Creator/1
  [EM_SoftECU_Transmit] -> Bus Creator/2
  [BAS_SoftECU_Transmit] -> Bus Creator/3
  [Engine_SoftECU_Transmit] -> Bus Creator/4
  Bus Creator/1 -> [From_ECUs]
  [GM_Transmit] -> Bus Creator/5
  [From_Supervisory] -> Subsystem/1(Supervisory)
  Subsystem/1(ESS) -> [ESS_SoftECU_Receive]
  Subsystem/2(EM) -> [EM_SoftECU_Receive]
  Subsystem/3(BAS) -> [BAS_SoftECU_Receive]
  Subsystem/4(ICE) -> [Engine_SoftECU_Receive]
  Subsystem/5(Super) -> [Supervisory_Receive]
  [From_GCM] -> Subsystem/2(GCM CAN), Subsystem1/1(From_GCM)
  Subsystem1/1(SoftECUPowerup) -> Subsystem/3(Relay Powerups)
  Subsystem1/2(MABxPowerup) -> Supervisory_Wakeup_Terminated/1
  Subsystem/6(Brusa) -> [Brusa_SoftECU_Receive]
  [Brusa_SoftECU_Transmit] -> Bus Creator/6
  Subsystem/7(CP1) -> [CP1_SoftECU_Receive]
  Subsystem/8(MShift) -> [Mastershift_SoftECU_Receive]
  [CP1_SoftECU_Transmit] -> Bus Creator/7
  [Mastershift_SoftECU_Transmit] -> Bus Creator/8
  Subsystem/9(Driver) -> [Driver_SoftECU_Receive]
  Subsystem/10(DCDC) -> [DCDC_SoftECU_Receive]
  [DCDC_SoftECU_Transmit] -> Bus Creator/9

== system EcoSIM3_P2_C2_WIP/Powertrain/Soft_ECUs_IO/VNT Kvaser ==
  CANRx : Subsystem
  CANTx : Subsystem
  ElectricalRx : Subsystem
  ElectricalTx : Subsystem
  Spine : Subsystem
  wires:
  ElectricalRx/1(Electrical) -> Spine/1(Electrical)
  CANRx/1(CAN Out) -> Spine/2(CAN)
  Spine/1(ElectricalTx) -> ElectricalTx/1(Electrical)
  Spine/2(CANTx) -> CANTx/1(CAN)

== system EcoSIM3_P2_C2_WIP/Powertrain/Soft_ECUs_IO/VNT Vector ==
  CANRx : Subsystem
  CANTx : Subsystem
  ElectricalRx : Subsystem
  ElectricalTx : Subsystem
  Spine : Subsystem
  wires:
  CANRx/1(CAN Out) -> Spine/2(CAN)
  Spine/1(ElectricalTx) -> ElectricalTx/1(Electrical)
  Spine/2(CANTx) -> CANTx/1(CAN)
  ElectricalRx/1(Electrical) -> Spine/1(Electrical)

== system EcoSIM3_P2_C2_WIP/Powertrain/Vehicle Dynamics/Sensor ==
  Bus Creator : BusCreator  Inputs=5
  Display : Display
  IVM : Subsystem
  Ideal Rotational Motion Sensor{,1..3} (4 alike) : fl_lib/Mechanical/Mechanical Sensors/Ideal Rotational Motion Sensor  offset=0 rad
  Mechanical Rotational Reference{,1..3} (4 alike) : fl_lib/Mechanical/Rotational Elements/Mechanical Rotational Reference
  PS-Simulink Converter{1..2,4..5} (4 alike) : nesl_utility/PS-Simulink Converter  PhysicalDomain=network_engine_domain  SubClassName=ps_output  LeftPortType=input  RightPortType=output  PseudoPeriodic=off  Frequencies=[]  Unit=rad  AffineConversion=off
  PS-Simulink Converter3 : nesl_utility/PS-Simulink Converter  PhysicalDomain=network_engine_domain  SubClassName=ps_output  LeftPortType=input  RightPortType=output  PseudoPeriodic=off  Frequencies=[]  Unit=m/s  AffineConversion=off
  Scope : Scope
      settings: SaveName=ScopeData75
  Sensor lag : Subsystem
  Sensor lag1 : Subsystem
  Sensor lag2 : Subsystem
  Sensor lag3 : Subsystem
  Sensor lag4 : Subsystem
  Vehicle_Speed : PMIOPort  Port=1  Side=Left
  FLT : PMIOPort  Port=2  Side=Left
  FRT : PMIOPort  Port=3  Side=Left
  RLT : PMIOPort  Port=4  Side=Right
  RRT : PMIOPort  Port=5  Side=Right
  Sensor_Out : Outport
  wires:
  PS-Simulink Converter3/1 -> Sensor lag/1(i)
  Sensor lag/1(o) -> IVM/1(mps), Bus Creator/1  "Vehicle_Speed_meter_per_s"
  PS-Simulink Converter1/1 -> Sensor lag1/1(i)
  PS-Simulink Converter2/1 -> Sensor lag2/1(i)
  PS-Simulink Converter4/1 -> Sensor lag3/1(i)
  PS-Simulink Converter5/1 -> Sensor lag4/1(i)
  Sensor lag1/1(o) -> Bus Creator/2  "Front_Left_Tire_Angle"
  Sensor lag3/1(o) -> Bus Creator/3  "Rear_Left_Tire_Angle"
  Sensor lag2/1(o) -> Bus Creator/4  "Front_Right_Tire_Angle"
  Sensor lag4/1(o) -> Bus Creator/5  "Rear_Right_Tire_Angle"
  Bus Creator/1 -> Sensor_Out/1
  IVM/1(Out1) -> Display/1, Scope/1
  connections:
  Vehicle_Speed/RConn1 -- PS-Simulink Converter3/LConn1
  Ideal Rotational Motion Sensor/LConn1 -- FLT/RConn1
  Ideal Rotational Motion Sensor1/LConn1 -- FRT/RConn1
  Ideal Rotational Motion Sensor/RConn1 -- Mechanical Rotational Reference/LConn1
  Ideal Rotational Motion Sensor2/RConn1 -- Mechanical Rotational Reference1/LConn1
  Ideal Rotational Motion Sensor3/RConn1 -- Mechanical Rotational Reference2/LConn1
  Ideal Rotational Motion Sensor1/RConn1 -- Mechanical Rotational Reference3/LConn1
  PS-Simulink Converter1/LConn1 -- Ideal Rotational Motion Sensor/RConn3
  PS-Simulink Converter2/LConn1 -- Ideal Rotational Motion Sensor1/RConn3
  Ideal Rotational Motion Sensor2/RConn3 -- PS-Simulink Converter4/LConn1
  PS-Simulink Converter5/LConn1 -- Ideal Rotational Motion Sensor3/RConn3
  RRT/RConn1 -- Ideal Rotational Motion Sensor3/LConn1
  RLT/RConn1 -- Ideal Rotational Motion Sensor2/LConn1

== system EcoSIM3_P2_C2_WIP/Powertrain/Vehicle Dynamics/Subsystem ==
  Ideal Force Sensor : fl_lib/Mechanical/Mechanical Sensors/Ideal Force Sensor
  R : PMIOPort  Port=1  Side=Right
  C : PMIOPort  Port=2  Side=Left
  F : PMIOPort  Port=3  Side=Left
  connections:
  Ideal Force Sensor/LConn1 -- R/RConn1
  Ideal Force Sensor/RConn1 -- C/RConn1
  F/RConn1 -- Ideal Force Sensor/RConn2

== system EcoSIM3_P2_C2_WIP/RTI Data/RTI Data Store/RTI Data Store ==
  RTI Data Store : Subsystem  mask(RTI_DATA_STORE){}
      mask help:
      | RTI Data Store Block. This block is used by RTI to store internal model dependent data. Deleting this block will result in data loss.
      |
      | NEVER DELETE, COPY, OR MODIFY THIS BLOCK!
      mask Help:
      | RTI Data Store Block. This block is used by RTI to store internal model dependent data. Deleting this block will result in data loss.
      | 
      | NEVER DELETE, COPY, OR MODIFY THIS BLOCK!
      mask Display: text(0.5, 0.5, ' ', 'HorizontalAlignment', 'center');

== system EcoSIM3_P2_C2_WIP/Supervisory Controller/Clutch Request/ClutchStatus ==
  In1 : Inport
  Add : Sum  Inputs=+++-
  Data Type Conversion : DataTypeConversion
  Data Type Conversion1 : DataTypeConversion
  Data Type Conversion2 : DataTypeConversion
  DisengagementThreshold : Constant  Value=6000
  EngagementThreshold : Constant  Value=100
  Gain1 : Gain  Gain=2
  Gain2 : Gain
  Gain3 : Gain  Gain=3
  Logical Operator : Logic  Operator=NOR  AllPortsSameDT=off  OutDataTypeStr=boolean
  Offset : Constant
  Relational Operator : RelationalOperator  Operator=<=  OutDataTypeStr=boolean
  Relational Operator1 : RelationalOperator  OutDataTypeStr=boolean
  Out1 : Outport
  wires:
  Gain2/1 -> Add/3
  Logical Operator/1 -> Data Type Conversion2/1
  In1/1 -> Relational Operator1/1, Relational Operator/1
  Relational Operator/1 -> Logical Operator/2, Data Type Conversion/1
  Data Type Conversion/1 -> Gain2/1
  Gain1/1 -> Add/1
  Gain3/1 -> Add/2
  Data Type Conversion1/1 -> Gain1/1
  EngagementThreshold/1 -> Relational Operator/2
  DisengagementThreshold/1 -> Relational Operator1/2
  Data Type Conversion2/1 -> Gain3/1
  Relational Operator1/1 -> Logical Operator/1, Data Type Conversion1/1
  Offset/1 -> Add/4
  Add/1 -> Out1/1

== system EcoSIM3_P2_C2_WIP/Supervisory Controller/Clutch Request/Signal Builder ==
  Demux : Demux  Tag=STV Demux  Outputs=1
  FromWs : FromWorkspace  Tag=STV FromWs  VariableName=tuvar  SampleTime=0
      SigBuilderData=|
      | common.afterFinalStr = 'Extrapolate'
      | common.sampleTime = 0
      | dataSet(1).timeRange = [0 10]
      | dataSet(1).name = 'Test1'
      | dataSet(2).timeRange = [0 232]
      | dataSet(2).name = 'OptimalReq'
      | dataSet(3).timeRange = [0 232]
      | dataSet(3).name = 'TrialReq'
      | sbobj.Groups(1).Name = 'Test1'
      | sbobj.Groups(1).Signals.Name = 'GearReq'
      | sbobj.Groups(1).Signals.XData = [0 0.01 0.02 0.03 0.04 0.05 0.06 0.07 0.08 0.09 0.1 0.11 ... (1001 elements, 1x1001)]
      | sbobj.Groups(1).Signals.YData = [1 1 1 1 1 1 1 1 1 1 1 1 ... (1001 elements, 1x1001)]
      | sbobj.Groups(2).Name = 'OptimalReq'
      | sbobj.Groups(2).Signals.Name = 'GearReq'
      | sbobj.Groups(2).Signals.XData = [0 0.01 0.02 0.03 0.04 0.05 0.06 0.07 0.08 0.09 0.1 0.11 ... (23201 elements, 1x23201)]
      | sbobj.Groups(2).Signals.YData = [1 1 1 1 1 1 1 1 1 1 1 1 ... (23201 elements, 1x23201)]
      | sbobj.Groups(2).TimeRange = [0 232]
      | sbobj.Groups(3).Name = 'TrialReq'
      | sbobj.Groups(3).Signals.Name = 'GearReq'
      | sbobj.Groups(3).Signals.XData = [0 0.01 0.02 0.03 0.04 0.05 0.06 0.07 0.08 0.09 0.1 0.11 ... (23201 elements, 1x23201)]
      | sbobj.Groups(3).Signals.YData = [1 1 1 1 1 1 1 1 1 1 1 1 ... (23201 elements, 1x23201)]
      | sbobj.Groups(3).TimeRange = [0 232]
  GearReq : Outport  Tag=STV Outport
  wires:
  Demux/1 -> GearReq/1
  FromWs/1 -> Demux/1

== system EcoSIM3_P2_C2_WIP/Supervisory Controller/Driver Requested Torque/Max Torque Calculation ==
  note: at the wheels
  Gear : Inport
  Engine Speed : Inport  Port=2
  Divide2 : Product  Inputs=**
  Max Torque : Lookup_n-D  NumberOfTableDimensions=1  BreakpointsForDimension1=Plants.ICE.Mdl.Plant.Max_Trq.w  Table=Plants.ICE.Mdl.Plant.Max_Trq.Trq  InternalRulePriority=Speed  RndMeth=Simplest  InputSameDT=on
  RearGR3 : Gain  Gain=2.77
  Scope : Scope  NumInputPorts=2
      settings: YMin=-5~-5  YMax=5~5  SaveName=ScopeData69
  TRAN GR2 : Lookup_n-D  NumberOfTableDimensions=1  BreakpointsForDimension1=Plants.Trans.Mdl.Plant.Gear_cmd  Table=Plants.Trans.Mdl.Plant.GR  ExtrapMethod=Clip  InternalRulePriority=Speed  RndMeth=Simplest  InputSameDT=on
  "Engine Torque " : Outport
  wires:
  TRAN GR2/1 -> Divide2/2
  Gear/1 -> TRAN GR2/1
  Engine Speed/1 -> Scope/1, Max Torque/1
  Divide2/1 -> "Engine Torque "/1
  Max Torque/1 -> Scope/2, RearGR3/1  "Engine Torque"
  RearGR3/1 -> Divide2/1

== system EcoSIM3_P2_C2_WIP/Supervisory Controller/Driver Requested Torque/Speed Calculations ==
  "Vehicle Speed m/s " : Inport
  Gear Current : Inport  Port=2
  Gain1 : Gain  Gain=2/Plants.Rear_wh.tire_diameter
  Gain2 : Gain  Gain=2.77
  Product : Product
  TRAN GR : Lookup_n-D  NumberOfTableDimensions=1  BreakpointsForDimension1=Plants.Trans.Mdl.Plant.Gear_cmd  Table=Plants.Trans.Mdl.Plant.GR  ExtrapMethod=Clip  InternalRulePriority=Speed  RndMeth=Simplest  InputSameDT=on
  Engine Speed : Outport
  "EM Speed " : Outport  Port=2
  wires:
  "Vehicle Speed m/s "/1 -> Gain1/1
  Gain2/1 -> "EM Speed "/1, Product/2
  Gain1/1 -> Gain2/1
  Product/1 -> Engine Speed/1
  Gear Current/1 -> TRAN GR/1
  TRAN GR/1 -> Product/1

== system EcoSIM3_P2_C2_WIP/Supervisory Controller/Functional Safety1/Functional Safety Algorithm ==
  Torque Requests : Inport
  ECU/Sensor Signals : Inport  Port=2
  Fault Detection (Team Developed) : Subsystem
  Fault Management : Subsystem
  Fault Mitigation : Subsystem
  Torque Limits : Outport
  Fault Code : Outport  Port=2
  wires:
  Torque Requests/1 -> Fault Detection (Team Developed)/1(Torque Requests)
  ECU/Sensor Signals/1 -> Fault Detection (Team Developed)/2(ECU/Sensor Signals), Fault Management/2(ECU/Sensor Signals)
  Fault Mitigation/1(Torque Limits) -> Torque Limits/1
  Fault Management/1(Fault Code) -> Fault Mitigation/1(Fault Code), Fault Code/1
  Fault Detection (Team Developed)/1(Team Dev Fault Signals) -> Fault Management/1(Team Dev Fault Signals)

== system EcoSIM3_P2_C2_WIP/Supervisory Controller/Input Conditioning/Alpha Conditioning ==
  Raw Alpha_V : Inport
  Add : Sum
  Bus Selector : BusSelector  OutputSignals=GM_Transmit.GM_Electrical_Out.Alpha_Low,GM_Transmit.GM_Electrical_Out.Alpha_High
  Constant : Constant  Value=0.4
  Constant1 : Constant  Value=0.8
  Output Scaling5 : Gain  Gain=50
  Output Scaling6 : Gain  Gain=25
  Output Scaling7 : Gain  Gain=0.5
  Scope : Scope
      settings: SaveName=ScopeData56
  Sum4 : Sum  Inputs=-+|
  Sum5 : Sum  Inputs=|+-
  Alpha Percent : Outport
  wires:
  Constant1/1 -> Sum5/2
  Sum5/1 -> Output Scaling6/1
  Output Scaling5/1 -> Add/1
  Output Scaling7/1 -> Scope/1, Alpha Percent/1  "Alpha_percent"
  Bus Selector/1 -> Sum4/2  "<Alpha_Low>"
  Output Scaling6/1 -> Add/2
  Constant/1 -> Sum4/1
  Add/1 -> Output Scaling7/1
  Sum4/1 -> Output Scaling5/1
  Bus Selector/2 -> Sum5/1  "<Alpha_High>"
  Raw Alpha_V/1 -> Bus Selector/1

== system EcoSIM3_P2_C2_WIP/Supervisory Controller/Input Conditioning/ModeSwitch Conditioning ==
  Bus Creator : BusCreator  Inputs=2
  Bus Selector : BusSelector  OutputSignals=DRIV_mode,Propulsion_mode
  Out1 : Outport
  wires:
  Bus Creator/1 -> Out1/1  "ModeSwitch_Conditioned"
  [Simulation_Parameters] -> Bus Selector/1
  Bus Selector/1 -> Bus Creator/1  "<DRIV_mode>"
  Bus Selector/2 -> Bus Creator/2  "<Propulsion_mode>"
